simulink model "gm_sampleModel61741_pp_47_1_sub"  (R2023b)
settings: Solver=VariableStepAuto  StartTime=0.0  StopTime=10.0  RelTol=1e-3
libraries: simulink x46, hdlsllib x1
(part 1 of 2)
settings Model: Creator=CW  LastModifiedBy=CW
settings OptimizationCC: BlockReduction=off  ConditionallyExecuteInputs=off
settings DebuggingCC: ArtificialAlgebraicLoopMsg=none  InheritedTsInSrcMsg=none

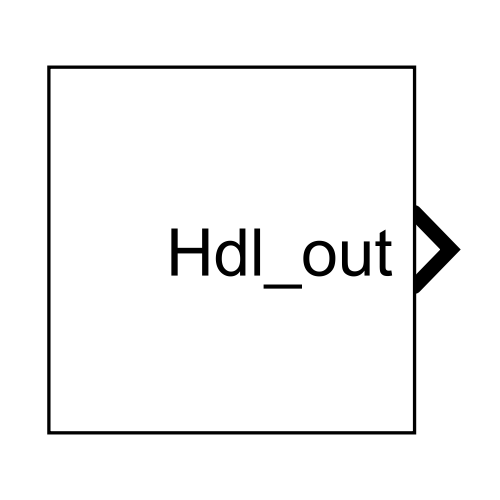
[thumbnail: Simulink's stored preview of the top-level diagram]
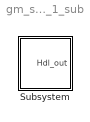
== system gm_sampleModel61741_pp_47_1_sub ==
  Subsystem : Subsystem

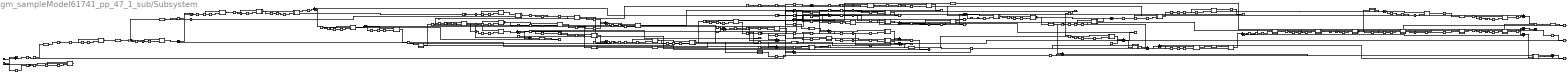
== system gm_sampleModel61741_pp_47_1_sub/Subsystem ==
  Reshape{,1..5} (6 alike) : Reshape
  cfblk1 : Subsystem  mask(Compare To Constant){relop=<=, const=double(3), OutDataTypeStr=uint8, ZeroCross=on}
      mask prompts: relop "Simulink:masks:Operator_MP"; const "Simulink:masks:ConstantValue_MP"; OutDataTypeStr "Simulink:masks:OutputDataType_MP"; ZeroCross "Simulink:masks:EnableZerocrossingDetection_MP"
      mask help: Simulink:masks:CompareToConstant_MD
      mask init:
      | OutDataTypeStr = 'uint8';
      | ZeroCross = 'on';
      | blkName = 'sampleModel61741_pp_47_1_sub/Subsystem/cfblk1';
      | const = double(3);
      | const_str = '3.0';
      | const_val = double(3);
      | relop = '<=';
      | setValue = 'fixdt(0, 8)';
      | str = '<= 3';
      mask TypeOptions relop: == | ~= | < | <= | >= | >
      mask TypeOptions OutDataTypeStr: Simulink:masks:uint8 | Simulink:masks:boolean
      mask Callback ZeroCross: sl('zeroCrossEnable', gcbh);
      mask Display: disp(str)
  cfblk{7,10,21,43,59,74,90,100,104,112,115,118,138,140,144,148} (16 alike) : Sum  OutDataTypeStr=uint8  AccumDataTypeStr=uint8  SampleTime=1
  cfblk{37,68,101,146} (4 alike) : MinMax  OutDataTypeStr=uint8
  cfblk{15..16,36,47,95,102,106,125,147} (9 alike) : Abs  SampleTime=1  OutDataTypeStr=uint8  SaturateOnIntegerOverflow=off
  cfblk103 : Subsystem
  cfblk{58,85,92,105} (4 alike) : Signum  SampleTime=1
  cfblk{18,73,93..94,107,131,145} (7 alike) : Sum  OutDataTypeStr=uint8  AccumDataTypeStr=uint8  RndMeth=Nearest  SampleTime=1
  cfblk107_const_val : Constant  Value=0  VectorParams1D=off  OutDataTypeStr=uint8  SampleTime=1
  cfblk109_inst : Subsystem
  cfblk11 : Sum  Inputs=+  OutDataTypeStr=uint8
  cfblk{22,27,39,44,61,69,86,110,128,137} (10 alike) : Sum  Inputs=+-  OutDataTypeStr=uint8  AccumDataTypeStr=uint8  SampleTime=1
  cfblk111 : Subsystem
  cfblk113 : Subsystem
  cfblk{20,24,35,54,57,91,114,134} (8 alike) : ComplexToRealImag  SampleTime=1
  cfblk{6,30,40,42,46,67,72,79..80,97,117,119,123} (13 alike) : Product  Inputs=*/  OutDataTypeStr=uint8  RndMeth=Zero  SaturateOnIntegerOverflow=on  SampleTime=1
  cfblk12 : Subsystem
  cfblk121 : Subsystem
  cfblk122 : Subsystem
  cfblk124 : Sum  Inputs=+  OutDataTypeStr=uint8
  cfblk126 : Subsystem  mask(Real World Value Increment){}
      mask help: Simulink:masks:RealWorldValueIncrement_MD
      mask Display: disp('V++')
  cfblk127 : Subsystem  mask(Real World Value Increment){}
      mask help: Simulink:masks:RealWorldValueIncrement_MD
      mask Display: disp('V++')
  cfblk13 : Subsystem
  cfblk130 : Subsystem
  cfblk131_const_val : Constant  Value=0  VectorParams1D=off  OutDataTypeStr=uint8  SampleTime=1
  cfblk132 : Subsystem
  cfblk133 : Subsystem
  cfblk135 : Subsystem
  cfblk139 : Subsystem
  cfblk14 : Subsystem
  cfblk141 : Subsystem  mask(Real World Value Increment){}
      mask help: Simulink:masks:RealWorldValueIncrement_MD
      mask Display: disp('V++')
  cfblk142 : Subsystem
  cfblk143_inst : Subsystem
  cfblk145_const_val : Constant  Value=0  VectorParams1D=off  OutDataTypeStr=uint8  SampleTime=1
  cfblk151 : Constant  OutDataTypeStr=uint8  SampleTime=1
  cfblk152 : Constant  OutDataTypeStr=uint8  SampleTime=1
  cfblk153 : hdlsllib/Sources/HDL Counter  CountType=Count limited  CountInit=0  CountStep=1  CountMax=25  CountFromType=Initial value  CountFrom=0  CountResetPort=off  CountLoadPort=off  CountEnbPort=off  CountDirPort=off  CountHitOutputPort=off  CountDataType=Unsigned  CountWordLen=8  CountFracLen=0  CountSampTime=1
  cfblk154 : Subsystem
  cfblk155 : Subsystem
  cfblk156 : Subsystem
  cfblk{157..160,162..171} (14 alike) : Delay  DelayLength=double(2)  InitialCondition=0  SampleTime=1
  cfblk17 : Gain  Gain="fi(0,0,8,7,\"hex\",\"80\")"  ParamDataTypeStr=fixdt(0, 8, 7)  OutDataTypeStr=uint8  SampleTime=1
  cfblk172 : Subsystem
  cfblk173 : DataTypeConversion  OutDataTypeStr=fixdt(0,8,0)
  cfblk174 : DataTypeConversion  OutDataTypeStr=fixdt(0,8,0)
  cfblk175 : Subsystem
  cfblk176 : Subsystem
  cfblk177 : Subsystem
  cfblk178 : DataTypeConversion  OutDataTypeStr=fixdt(0,8,0)
  cfblk18_const_val : Constant  Value=0  VectorParams1D=off  OutDataTypeStr=uint8  SampleTime=1
  cfblk19 : Subsystem
  cfblk2 : Subsystem  mask(Compare To Constant){relop=<=, const=double(3), OutDataTypeStr=uint8, ZeroCross=on}
      mask prompts: relop "Simulink:masks:Operator_MP"; const "Simulink:masks:ConstantValue_MP"; OutDataTypeStr "Simulink:masks:OutputDataType_MP"; ZeroCross "Simulink:masks:EnableZerocrossingDetection_MP"
      mask help: Simulink:masks:CompareToConstant_MD
      mask init:
      | OutDataTypeStr = 'uint8';
      | ZeroCross = 'on';
      | blkName = 'sampleModel61741_pp_47_1_sub/Subsystem/cfblk2';
      | const = double(3);
      | const_str = '3.0';
      | const_val = double(3);
      | relop = '<=';
      | setValue = 'fixdt(0, 8)';
      | str = '<= 3';
      mask TypeOptions relop: == | ~= | < | <= | >= | >
      mask TypeOptions OutDataTypeStr: Simulink:masks:uint8 | Simulink:masks:boolean
      mask Callback ZeroCross: sl('zeroCrossEnable', gcbh);
      mask Display: disp(str)
  cfblk23 : Subsystem
  cfblk26 : Subsystem
  cfblk28 : Subsystem
  cfblk29 : Sum  Inputs=+  OutDataTypeStr=uint8
  cfblk3 : simulink/Logic and Bit Operations/Detect Change  vinit=0  OutDataTypeStr=uint8
      settings: LibrarySourceBlock=|
      | hdlsllib/Logic and Bit
      | Operations/Detect
      | Change
  cfblk31_inst : Subsystem
  cfblk32 : Subsystem
  cfblk33 : Subsystem
  cfblk34 : Subsystem  mask(Real World Value Increment){}
      mask help: Simulink:masks:RealWorldValueIncrement_MD
      mask Display: disp('V++')
  cfblk38 : Subsystem  mask(Real World Value Increment){}
      mask help: Simulink:masks:RealWorldValueIncrement_MD
      mask Display: disp('V++')
  cfblk4 : Subsystem  mask(Detect Rise Nonnegative){vinit=double(0), InputProcessing=Elements as channels (sample based), OutDataTypeStr=uint8}
      mask prompts: vinit "Simulink:masks:InitialCondition_MP"; InputProcessing "Simulink:masks:InputProcessing_MP"; OutDataTypeStr "Simulink:masks:OutputDataType_MP"
      mask help: Simulink:masks:DetectRiseNonnegative_MD
      mask init:
      | InputProcessing = 'Elements as channels (sample based)';
      | OutDataTypeStr = 'uint8';
      | vinit = double(0);
      mask TypeOptions InputProcessing: Simulink:masks:ColumnsAsChannelsFrameBased | Simulink:masks:ElementsAsChannelsSampleBased
      mask TypeOptions OutDataTypeStr: Simulink:masks:uint8 | Simulink:masks:boolean
      mask Display: fprintf('U >= 0\n&  NOT\nU/z >= 0')
  cfblk41 : Subsystem
  cfblk45 : Subsystem  mask(Real World Value Increment){}
      mask help: Simulink:masks:RealWorldValueIncrement_MD
      mask Display: disp('V++')
  cfblk48 : Subsystem
  cfblk49 : Subsystem  mask(Real World Value Increment){}
      mask help: Simulink:masks:RealWorldValueIncrement_MD
      mask Display: disp('V++')
  cfblk5 : simulink/Logic and Bit Operations/Detect Decrease  vinit=0.0  OutDataTypeStr=uint8
      settings: LibrarySourceBlock=|
      | hdlsllib/Logic and Bit
      | Operations/Detect
      | Decrease
  cfblk50_inst : Subsystem
  cfblk51 : Subsystem
  cfblk55 : Subsystem
  cfblk56 : Subsystem
  cfblk60 : Subsystem
  cfblk62 : Subsystem
  cfblk63 : Subsystem  mask(Real World Value Increment){}
      mask help: Simulink:masks:RealWorldValueIncrement_MD
      mask Display: disp('V++')
  cfblk64 : Subsystem
  cfblk65 : Subsystem
  cfblk66 : Subsystem
  cfblk71 : Subsystem
  cfblk73_const_val : Constant  Value=0  VectorParams1D=off  OutDataTypeStr=uint8  SampleTime=1
  cfblk75 : Subsystem  mask(Real World Value Increment){}
      mask help: Simulink:masks:RealWorldValueIncrement_MD
      mask Display: disp('V++')
  cfblk76 : Subsystem
  cfblk77 : Subsystem
  cfblk78 : Subsystem
  cfblk8 : Subsystem
  cfblk81 : Subsystem
  cfblk82 : Subsystem
  cfblk83_inst : Subsystem
  cfblk87 : Subsystem
  cfblk9 : Gain  Gain="fi(0,0,8,7,\"hex\",\"80\")"  ParamDataTypeStr=fixdt(0, 8, 7)  OutDataTypeStr=uint8  SampleTime=1
  cfblk93_const_val : Constant  Value=0  VectorParams1D=off  OutDataTypeStr=uint8  SampleTime=1
  cfblk94_const_val : Constant  Value=0  VectorParams1D=off  OutDataTypeStr=uint8  SampleTime=1
  cfblk96_inst : Subsystem
  cfblk98 : Subsystem
  cfblk99 : Gain  Gain="fi(0,0,8,7,\"hex\",\"80\")"  ParamDataTypeStr=fixdt(0, 8, 7)  OutDataTypeStr=uint8  SampleTime=1
  compare{,2,7..8,14..16,23,25,32..33,35..36} (13 alike) : simulink/Logic and Bit Operations/Compare To Constant  relop=>=  const=0  OutDataTypeStr=boolean
  compare{1,3..4,6,9..13,17..20,22,26..27,30..31,34,37..38,40,42..43} (24 alike) : simulink/Logic and Bit Operations/Compare To Constant  relop=>=  const=255  OutDataTypeStr=boolean
  compare21 : simulink/Logic and Bit Operations/Compare To Constant  relop=>=  const=3  OutDataTypeStr=boolean
  compare24 : simulink/Logic and Bit Operations/Compare To Constant  relop=>=  const=2  OutDataTypeStr=boolean
  compare28 : simulink/Logic and Bit Operations/Compare To Constant  relop=>=  const=3  OutDataTypeStr=boolean
  compare{5,29,39,41} (4 alike) : simulink/Logic and Bit Operations/Compare To Constant  relop=>=  const=1  OutDataTypeStr=boolean
  emi_{6,14,23,31,39,47,55,63,71,79,87,95,103,111,120,128,136,144,152,161,169,177,186,194,202,210,218,227,235,244,252,261,269,277,285,293,309,317,325,333,341,349,357,365} (44 alike) : DataTypeConversion  OutDataTypeStr=fixdt(0,8,0)
  emi_{24,40,48,104,121,153,162,211,219,278,294,350,358} (13 alike) : Delay  DelayLength=double(2)  InitialCondition=0  SampleTime=1
  emi_{7,15,32,56,72,88,96,112,129,145,170,178,187,195,203,228,236,245,253,270,310,334,342,366} (24 alike) : Delay  DelayLength=double(2)  InitialCondition=255  SampleTime=1
  emi_{64,80,137,326} (4 alike) : Delay  DelayLength=double(2)  InitialCondition=1  SampleTime=1
  emi_262 : Delay  DelayLength=double(2)  InitialCondition=3  SampleTime=1
  emi_286 : Delay  DelayLength=double(2)  InitialCondition=2  SampleTime=1
  emi_318 : Delay  DelayLength=double(2)  InitialCondition=3  SampleTime=1
  Hdl_out : Outport  OutDataTypeStr=uint8  SampleTime=1
  wires:
  cfblk1/1(y) -> cfblk17/1
  cfblk10/1 -> cfblk22/1, cfblk80/2
  cfblk100/1 -> Hdl_out/1, cfblk155/1(In1)
  cfblk101/1 -> cfblk140/2
  cfblk102/1 -> emi_245/1, cfblk55/1(emi_238)
  cfblk103/1(emi_2) -> cfblk10/2
  cfblk104/1 -> cfblk138/2, cfblk115/1
  cfblk105/1 -> cfblk90/2, emi_112/1, cfblk139/1(emi_106)
  cfblk106/1 -> emi_278/1, cfblk172/1(emi_272)
  cfblk107/1 -> Reshape5/1
  cfblk109_inst/1(out1) -> cfblk148/2
  cfblk11/1 -> cfblk75/1(u)
  cfblk110/1 -> cfblk119/1
  cfblk111/1(emi_156) -> cfblk163/1
  cfblk111/2(emi_157) -> cfblk69/1, cfblk167/1
  cfblk112/1 -> emi_318/1, cfblk76/1(emi_312)
  cfblk113/1(emi_18) -> cfblk110/1
  cfblk113/2(emi_19) -> cfblk100/1
  cfblk114/1 -> cfblk5/1
  cfblk114/2 -> cfblk109_inst/1(in1)
  cfblk115/1 -> cfblk74/2
  Reshape/1 -> emi_342/1, cfblk82/1(emi_336)
  cfblk117/1 -> cfblk128/2, cfblk102/1, cfblk100/2
  cfblk118/1 -> emi_162/1, cfblk111/1(emi_155)
  cfblk119/1 -> cfblk162/1
  cfblk12/1(emi_35) -> emi_24/1, cfblk113/1(emi_17)
  Reshape1/1 -> emi_104/1, cfblk135/1(emi_98)
  cfblk121/1(emi_43) -> cfblk118/1
  cfblk122/1(emi_51) -> emi_145/1, cfblk98/1(emi_139)
  cfblk123/1 -> cfblk93/1
  cfblk124/1 -> cfblk72/2
  cfblk125/1 -> emi_170/1, cfblk19/1(emi_164), cfblk97/2
  cfblk126/1(y) -> cfblk86/1
  cfblk127/1(y) -> cfblk85/1, cfblk117/2
  cfblk128/1 -> emi_72/1, cfblk13/1(emi_66)
  cfblk13/1(emi_67) -> cfblk110/2
  cfblk130/1(emi_75) -> emi_137/1, cfblk175/1(emi_131)
  cfblk131/1 -> cfblk104/2, emi_326/1, cfblk78/1(emi_320)
  cfblk132/1(emi_83) -> emi_129/1, cfblk142/1(emi_123)
  cfblk133/1(emi_91) -> emi_270/1, cfblk62/1(emi_264)
  cfblk134/1 -> cfblk21/1
  cfblk134/2 -> cfblk90/1
  cfblk135/1(emi_99) -> cfblk44/2
  cfblk137/1 -> emi_334/1, cfblk8/1(emi_328)
  cfblk138/1 -> cfblk123/2
  cfblk139/1(emi_107) -> emi_253/1, cfblk56/1(emi_247)
  cfblk14/1(emi_115) -> cfblk173/1
  cfblk14/2(emi_116) -> cfblk174/1
  cfblk140/1 -> emi_178/1, cfblk23/1(emi_172)
  cfblk141/1(y) -> cfblk128/1
  cfblk142/1(emi_124) -> cfblk38/1(u), cfblk42/2
  cfblk143_inst/1(out1) -> cfblk59/1
  cfblk144/1 -> cfblk97/1
  cfblk145/1 -> cfblk95/1
  cfblk146/1 -> cfblk115/2
  cfblk147/1 -> cfblk165/1
  cfblk148/1 -> cfblk159/1
  cfblk15/1 -> cfblk158/1
  cfblk151/1 -> cfblk24/1
  cfblk152/1 -> cfblk131/1
  cfblk153/1 -> cfblk43/2, cfblk43/1, Reshape1/1
  cfblk154/1(emi_361) -> cfblk105/1
  cfblk155/1(Out1) -> Reshape2/1
  cfblk156/1(Out1) -> cfblk143_inst/1(in1)
  cfblk157/1 -> cfblk40/2
  cfblk158/1 -> cfblk79/2
  cfblk159/1 -> cfblk39/1
  cfblk16/1 -> cfblk137/1
  cfblk160/1 -> cfblk59/2
  cfblk162/1 -> cfblk83_inst/2(in2)
  cfblk163/1 -> cfblk42/1
  cfblk164/1 -> cfblk27/1
  cfblk165/1 -> cfblk10/1
  cfblk166/1 -> cfblk118/2
  cfblk167/1 -> cfblk138/1
  cfblk168/1 -> cfblk61/2
  cfblk169/1 -> cfblk80/1
  cfblk17/1 -> emi_64/1, cfblk81/1(emi_58)
  cfblk170/1 -> cfblk7/1
  cfblk171/1 -> cfblk30/2
  cfblk172/1(emi_273) -> cfblk54/1
  cfblk173/1 -> cfblk7/2
  cfblk174/1 -> emi_211/1, cfblk177/1(emi_205)
  cfblk175/1(emi_132) -> emi_121/1, cfblk14/1(emi_114)
  cfblk176/1(emi_148) -> cfblk67/2, cfblk29/1
  cfblk177/1(emi_206) -> cfblk50_inst/1(in1)
  cfblk178/1 -> cfblk50_inst/2(in2)
  cfblk18/1 -> cfblk148/1
  cfblk19/1(emi_165) -> cfblk134/1
  cfblk2/1(y) -> cfblk157/1
  cfblk20/1 -> Reshape3/1
  cfblk20/2 -> cfblk169/1, cfblk46/2
  cfblk21/1 -> cfblk44/1
  cfblk22/1 -> cfblk2/1(u)
  cfblk23/1(emi_173) -> cfblk127/1(u)
  cfblk24/1 -> cfblk35/1
  cfblk24/2 -> cfblk144/1
  Reshape2/1 -> cfblk96_inst/1(in1)
  cfblk26/1(emi_10) -> cfblk73/1
  cfblk27/1 -> emi_350/1, cfblk87/1(emi_344)
  cfblk28/1(emi_231) -> cfblk11/1
  cfblk29/1 -> cfblk140/1
  cfblk3/1 -> cfblk160/1
  cfblk30/1 -> cfblk57/1, emi_310/1, cfblk99/1, cfblk71/1(emi_304)
  cfblk31_inst/1(out1) -> cfblk168/1, cfblk6/2
  cfblk32/1(emi_181) -> cfblk171/1
  cfblk32/2(emi_182) -> cfblk69/2
  cfblk33/1(emi_353) -> emi_294/1, cfblk65/1(emi_288)
  cfblk34/1(y) -> cfblk18/1, cfblk9/1
  cfblk35/1 -> cfblk16/1
  cfblk35/2 -> cfblk36/1
  cfblk36/1 -> cfblk141/1(u)
  cfblk37/1 -> cfblk117/1
  cfblk38/1(y) -> cfblk146/1
  cfblk39/1 -> emi_195/1, cfblk41/1(emi_189)
  cfblk4/1(Y) -> cfblk178/1, cfblk124/1
  cfblk40/1 -> emi_32/1, cfblk77/1(emi_26)
  cfblk41/1(emi_190) -> cfblk156/1(In1)
  cfblk42/1 -> emi_228/1, cfblk51/1(emi_221)
  cfblk43/1 -> cfblk123/1
  cfblk44/1 -> cfblk15/1
  cfblk45/1(y) -> cfblk63/1(u)
  cfblk46/1 -> cfblk145/1
  cfblk47/1 -> cfblk144/2
  cfblk48/1(emi_214) -> cfblk1/1(u), cfblk4/1(U)
  cfblk49/1(y) -> cfblk21/2
  cfblk5/1 -> cfblk58/1
  cfblk50_inst/1(out1) -> emi_153/1, cfblk176/1(emi_147)
  cfblk51/1(emi_222) -> cfblk49/1(u)
  cfblk51/2(emi_223) -> cfblk20/1
  Reshape3/1 -> cfblk104/1, emi_40/1, cfblk12/1(emi_34)
  cfblk54/1 -> cfblk107/1
  cfblk54/2 -> cfblk68/1
  cfblk55/1(emi_239) -> cfblk170/1
  cfblk56/1(emi_248) -> emi_56/1, cfblk122/1(emi_50), cfblk126/1(u)
  cfblk57/1 -> cfblk31_inst/2(in2)
  cfblk57/2 -> cfblk22/2
  cfblk58/1 -> emi_219/1, cfblk48/1(emi_213)
  cfblk59/1 -> emi_366/1, cfblk154/1(emi_360)
  cfblk6/1 -> emi_203/1, cfblk66/1(emi_197)
  cfblk60/1(emi_256) -> cfblk92/1
  cfblk60/2(emi_257) -> cfblk86/2
  cfblk61/1 -> cfblk72/1
  cfblk62/1(emi_265) -> cfblk91/1
  cfblk63/1(y) -> cfblk46/1
  cfblk64/1(emi_281) -> cfblk112/2
  cfblk65/1(emi_289) -> cfblk112/1, cfblk34/1(u)
  cfblk66/1(emi_198) -> cfblk94/1
  cfblk67/1 -> emi_88/1, cfblk132/1(emi_82)
  cfblk68/1 -> cfblk106/1
  cfblk69/1 -> emi_358/1, cfblk33/1(emi_352)
  cfblk7/1 -> cfblk40/1
  cfblk71/1(emi_305) -> emi_96/1, emi_7/1, cfblk103/1(emi_1), cfblk133/1(emi_90)
  cfblk72/1 -> emi_80/1, cfblk130/1(emi_74)
  cfblk73/1 -> cfblk67/1
  cfblk74/1 -> cfblk39/2
  cfblk75/1(y) -> Reshape/1
  cfblk76/1(emi_313) -> Reshape4/1
  cfblk77/1(emi_27) -> cfblk27/2
  cfblk78/1(emi_321) -> cfblk37/1
  cfblk79/1 -> cfblk83_inst/1(in1)
  cfblk8/1(emi_329) -> emi_187/1, cfblk32/1(emi_180)
  cfblk80/1 -> emi_15/1, cfblk26/1(emi_9)
  cfblk81/1(emi_59) -> cfblk61/1
  cfblk82/1(emi_337) -> cfblk47/1
  cfblk83_inst/1(out1) -> cfblk30/1
  Reshape4/1 -> emi_262/1, cfblk60/1(emi_255)
  cfblk85/1 -> cfblk119/2
  cfblk86/1 -> emi_236/1, cfblk28/1(emi_230)
  cfblk87/1(emi_345) -> cfblk79/1
  Reshape5/1 -> cfblk114/1
  cfblk9/1 -> cfblk147/1, cfblk143_inst/2(in2), emi_286/1, cfblk64/1(emi_280), cfblk6/1
  cfblk90/1 -> cfblk109_inst/2(in2)
  cfblk91/1 -> cfblk101/1
  cfblk91/2 -> cfblk45/1(u)
  cfblk92/1 -> cfblk164/1
  cfblk93/1 -> emi_48/1, cfblk121/1(emi_42)
  cfblk94/1 -> cfblk96_inst/2(in2), cfblk166/1
  cfblk95/1 -> cfblk31_inst/1(in1)
  cfblk96_inst/1(out1) -> cfblk74/1
  cfblk97/1 -> cfblk3/1
  cfblk98/1(emi_140) -> cfblk125/1
  cfblk99/1 -> cfblk137/2
  emi_103/1 -> compare/1
  emi_104/1 -> emi_103/1
  emi_111/1 -> compare1/1
  emi_112/1 -> emi_111/1
  emi_120/1 -> compare2/1
  emi_121/1 -> emi_120/1
  emi_128/1 -> compare3/1
  emi_129/1 -> emi_128/1
  emi_136/1 -> compare5/1
  emi_137/1 -> emi_136/1
  emi_14/1 -> compare4/1
  emi_144/1 -> compare6/1
  emi_145/1 -> emi_144/1
  emi_15/1 -> emi_14/1
  emi_152/1 -> compare7/1
  emi_153/1 -> emi_152/1
  emi_161/1 -> compare8/1
  emi_162/1 -> emi_161/1
  emi_169/1 -> compare9/1
  emi_170/1 -> emi_169/1
  emi_177/1 -> compare10/1
  emi_178/1 -> emi_177/1
  emi_186/1 -> compare11/1
  emi_187/1 -> emi_186/1
  emi_194/1 -> compare12/1
  emi_195/1 -> emi_194/1
  emi_202/1 -> compare13/1
  emi_203/1 -> emi_202/1
  emi_210/1 -> compare14/1
  emi_211/1 -> emi_210/1
  emi_218/1 -> compare15/1
  emi_219/1 -> emi_218/1
  emi_227/1 -> compare17/1
  emi_228/1 -> emi_227/1
  emi_23/1 -> compare16/1
  emi_235/1 -> compare18/1
  emi_236/1 -> emi_235/1
  emi_24/1 -> emi_23/1
  emi_244/1 -> compare19/1
  emi_245/1 -> emi_244/1
  emi_252/1 -> compare20/1
  emi_253/1 -> emi_252/1
  emi_261/1 -> compare21/1
  emi_262/1 -> emi_261/1
  emi_269/1 -> compare22/1
  emi_270/1 -> emi_269/1
  emi_277/1 -> compare23/1
  emi_278/1 -> emi_277/1
  emi_285/1 -> compare24/1
  emi_286/1 -> emi_285/1
  emi_293/1 -> compare25/1
  emi_294/1 -> emi_293/1
  emi_309/1 -> compare27/1
  emi_31/1 -> compare26/1
  emi_310/1 -> emi_309/1
  emi_317/1 -> compare28/1
  emi_318/1 -> emi_317/1
  emi_32/1 -> emi_31/1
  emi_325/1 -> compare29/1
  emi_326/1 -> emi_325/1
  emi_333/1 -> compare30/1
  emi_334/1 -> emi_333/1
  emi_341/1 -> compare31/1
  emi_342/1 -> emi_341/1
  emi_349/1 -> compare32/1
  emi_350/1 -> emi_349/1
  emi_357/1 -> compare33/1
  emi_358/1 -> emi_357/1
  emi_365/1 -> compare34/1
  emi_366/1 -> emi_365/1
  emi_39/1 -> compare35/1
  emi_40/1 -> emi_39/1
  emi_47/1 -> compare36/1
  emi_48/1 -> emi_47/1
  emi_55/1 -> compare38/1
  emi_56/1 -> emi_55/1
  emi_6/1 -> compare37/1
  emi_63/1 -> compare39/1
  emi_64/1 -> emi_63/1
  emi_7/1 -> emi_6/1
  emi_71/1 -> compare40/1
  emi_72/1 -> emi_71/1
  emi_79/1 -> compare41/1
  emi_80/1 -> emi_79/1
  emi_87/1 -> compare42/1
  emi_88/1 -> emi_87/1
  emi_95/1 -> compare43/1
  emi_96/1 -> emi_95/1
  cfblk107_const_val/1 -> cfblk107/2
  cfblk131_const_val/1 -> cfblk131/2
  cfblk145_const_val/1 -> cfblk145/2
  cfblk18_const_val/1 -> cfblk18/2
  cfblk73_const_val/1 -> cfblk73/2
  cfblk93_const_val/1 -> cfblk93/2
  cfblk94_const_val/1 -> cfblk94/2
  compare/1 -> cfblk135/2(Action Port)
  compare1/1 -> cfblk139/2(Action Port)
  compare2/1 -> cfblk14/2(Action Port)
  compare3/1 -> cfblk142/2(Action Port)
  compare4/1 -> cfblk26/2(Action Port)
  compare5/1 -> cfblk175/2(Action Port)
  compare6/1 -> cfblk98/2(Action Port)
  compare7/1 -> cfblk176/2(Action Port)
  compare8/1 -> cfblk111/2(Action Port)
  compare9/1 -> cfblk19/2(Action Port)
  compare10/1 -> cfblk23/2(Action Port)
  compare11/1 -> cfblk32/2(Action Port)
  compare12/1 -> cfblk41/2(Action Port)
  compare13/1 -> cfblk66/2(Action Port)
  compare14/1 -> cfblk177/2(Action Port)
  compare15/1 -> cfblk48/2(Action Port)
  compare16/1 -> cfblk113/2(Action Port)
  compare17/1 -> cfblk51/2(Action Port)
  compare18/1 -> cfblk28/2(Action Port)
  compare19/1 -> cfblk55/2(Action Port)
  compare20/1 -> cfblk56/2(Action Port)
  compare21/1 -> cfblk60/2(Action Port)
  compare22/1 -> cfblk62/2(Action Port)
  compare23/1 -> cfblk172/2(Action Port)
  compare24/1 -> cfblk64/2(Action Port)
  compare25/1 -> cfblk65/2(Action Port)
  compare26/1 -> cfblk77/2(Action Port)
  compare27/1 -> cfblk71/2(Action Port)
  compare28/1 -> cfblk76/2(Action Port)
  compare29/1 -> cfblk78/2(Action Port)
  compare30/1 -> cfblk8/2(Action Port)
  compare31/1 -> cfblk82/2(Action Port)
  compare32/1 -> cfblk87/2(Action Port)
  compare33/1 -> cfblk33/2(Action Port)
  compare34/1 -> cfblk154/2(Action Port)
  compare35/1 -> cfblk12/2(Action Port)
  compare36/1 -> cfblk121/2(Action Port)
  compare37/1 -> cfblk103/2(Action Port)
  compare38/1 -> cfblk122/2(Action Port)
  compare39/1 -> cfblk81/2(Action Port)
  compare40/1 -> cfblk13/2(Action Port)
  compare41/1 -> cfblk130/2(Action Port)
  compare42/1 -> cfblk132/2(Action Port)
  compare43/1 -> cfblk133/2(Action Port)

== system gm_sampleModel61741_pp_47_1_sub/Subsystem/cfblk1 ==
  u : Inport  OutDataTypeStr=uint8  SampleTime=1
  Compare : RelationalOperator  Operator=<=  OutDataTypeStr=fixdt(0, 8)
  Constant : Constant  DisableCoverage=on  Value=const  OutDataTypeStr=Inherit: Inherit via back propagation  SampleTime=-1
  y : Outport  SampleTime=1
  wires:
  u/1 -> Compare/1
  Compare/1 -> y/1
  Constant/1 -> Compare/2

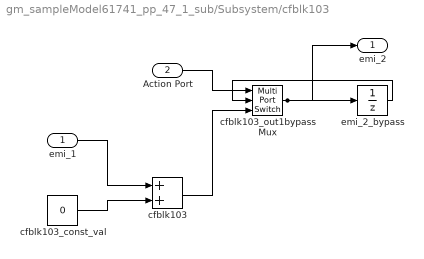
== system gm_sampleModel61741_pp_47_1_sub/Subsystem/cfblk103 ==
  emi_1 : Inport  OutDataTypeStr=uint8  PortDimensions=1  SampleTime=1
  Action Port : Inport  Port=2  OutDataTypeStr=boolean  SampleTime=1
  cfblk103 : Sum  OutDataTypeStr=uint8  AccumDataTypeStr=uint8  RndMeth=Nearest  SampleTime=1
  cfblk103_const_val : Constant  Value=0  VectorParams1D=off  OutDataTypeStr=uint8  SampleTime=1
  cfblk103_out1bypassMux : MultiPortSwitch  DataPortOrder=Zero-based contiguous  Inputs=2  zeroidx=on  OutDataTypeStr=uint8  SampleTime=1  SaturateOnIntegerOverflow=off  InputSameDT=off
  emi_2_bypass : UnitDelay  InitialCondition="fi(0,0,8,0,\"hex\",\"00\")"  SampleTime=1
  emi_2 : Outport  SampleTime=1  InitialOutput=0
  wires:
  Action Port/1 -> cfblk103_out1bypassMux/1
  emi_1/1 -> cfblk103/1
  cfblk103/1 -> cfblk103_out1bypassMux/3
  cfblk103_out1bypassMux/1 -> emi_2_bypass/1, emi_2/1
  emi_2_bypass/1 -> cfblk103_out1bypassMux/2
  cfblk103_const_val/1 -> cfblk103/2

== system gm_sampleModel61741_pp_47_1_sub/Subsystem/cfblk109_inst ==
  in1 : Inport  OutDataTypeStr=uint8  SampleTime=1
  in2 : Inport  Port=2  OutDataTypeStr=uint8  SampleTime=1
  mul_cfblk109_dotp_mulcomp : Product  Inputs=**  OutDataTypeStr=uint8  SampleTime=1
  out1 : Outport  OutDataTypeStr=uint8  SampleTime=1
  wires:
  in1/1 -> mul_cfblk109_dotp_mulcomp/1
  in2/1 -> mul_cfblk109_dotp_mulcomp/2
  mul_cfblk109_dotp_mulcomp/1 -> out1/1

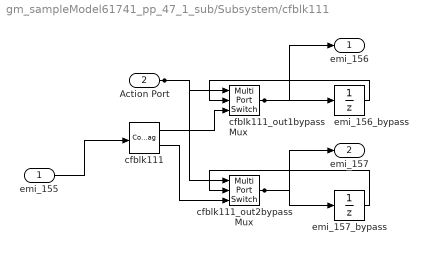
== system gm_sampleModel61741_pp_47_1_sub/Subsystem/cfblk111 ==
  emi_155 : Inport  OutDataTypeStr=uint8  PortDimensions=1  SampleTime=1
  Action Port : Inport  Port=2  OutDataTypeStr=boolean  SampleTime=1
  cfblk111 : ComplexToRealImag  SampleTime=1
  cfblk111_out1bypassMux : MultiPortSwitch  DataPortOrder=Zero-based contiguous  Inputs=2  zeroidx=on  OutDataTypeStr=uint8  SampleTime=1  SaturateOnIntegerOverflow=off  InputSameDT=off
  cfblk111_out2bypassMux : MultiPortSwitch  DataPortOrder=Zero-based contiguous  Inputs=2  zeroidx=on  OutDataTypeStr=uint8  SampleTime=1  SaturateOnIntegerOverflow=off  InputSameDT=off
  emi_156_bypass : UnitDelay  InitialCondition="fi(0,0,8,0,\"hex\",\"00\")"  SampleTime=1
  emi_157_bypass : UnitDelay  InitialCondition="fi(0,0,8,0,\"hex\",\"00\")"  SampleTime=1
  emi_156 : Outport  SampleTime=1  InitialOutput=0
  emi_157 : Outport  Port=2  SampleTime=1  InitialOutput=0
  wires:
  Action Port/1 -> cfblk111_out2bypassMux/1, cfblk111_out1bypassMux/1
  emi_155/1 -> cfblk111/1
  cfblk111/1 -> cfblk111_out1bypassMux/3
  cfblk111/2 -> cfblk111_out2bypassMux/3
  cfblk111_out1bypassMux/1 -> emi_156_bypass/1, emi_156/1
  emi_156_bypass/1 -> cfblk111_out1bypassMux/2
  cfblk111_out2bypassMux/1 -> emi_157_bypass/1, emi_157/1
  emi_157_bypass/1 -> cfblk111_out2bypassMux/2

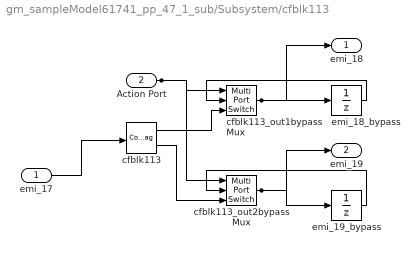
== system gm_sampleModel61741_pp_47_1_sub/Subsystem/cfblk113 ==
  emi_17 : Inport  OutDataTypeStr=uint8  PortDimensions=1  SampleTime=1
  Action Port : Inport  Port=2  OutDataTypeStr=boolean  SampleTime=1
  cfblk113 : ComplexToRealImag  SampleTime=1
  cfblk113_out1bypassMux : MultiPortSwitch  DataPortOrder=Zero-based contiguous  Inputs=2  zeroidx=on  OutDataTypeStr=uint8  SampleTime=1  SaturateOnIntegerOverflow=off  InputSameDT=off
  cfblk113_out2bypassMux : MultiPortSwitch  DataPortOrder=Zero-based contiguous  Inputs=2  zeroidx=on  OutDataTypeStr=uint8  SampleTime=1  SaturateOnIntegerOverflow=off  InputSameDT=off
  emi_18_bypass : UnitDelay  InitialCondition="fi(0,0,8,0,\"hex\",\"00\")"  SampleTime=1
  emi_19_bypass : UnitDelay  InitialCondition="fi(0,0,8,0,\"hex\",\"00\")"  SampleTime=1
  emi_18 : Outport  SampleTime=1  InitialOutput=0
  emi_19 : Outport  Port=2  SampleTime=1  InitialOutput=0
  wires:
  Action Port/1 -> cfblk113_out2bypassMux/1, cfblk113_out1bypassMux/1
  emi_17/1 -> cfblk113/1
  cfblk113/1 -> cfblk113_out1bypassMux/3
  cfblk113/2 -> cfblk113_out2bypassMux/3
  cfblk113_out1bypassMux/1 -> emi_18_bypass/1, emi_18/1
  emi_18_bypass/1 -> cfblk113_out1bypassMux/2
  cfblk113_out2bypassMux/1 -> emi_19_bypass/1, emi_19/1
  emi_19_bypass/1 -> cfblk113_out2bypassMux/2

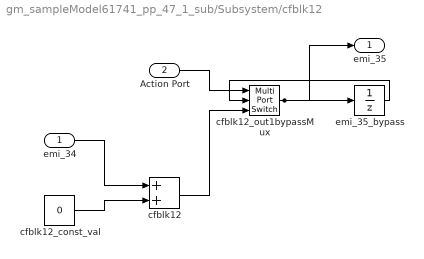
== system gm_sampleModel61741_pp_47_1_sub/Subsystem/cfblk12 ==
  emi_34 : Inport  OutDataTypeStr=uint8  PortDimensions=1  SampleTime=1
  Action Port : Inport  Port=2  OutDataTypeStr=boolean  SampleTime=1
  cfblk12 : Sum  OutDataTypeStr=uint8  AccumDataTypeStr=uint8  RndMeth=Nearest  SampleTime=1
  cfblk12_const_val : Constant  Value=0  VectorParams1D=off  OutDataTypeStr=uint8  SampleTime=1
  cfblk12_out1bypassMux : MultiPortSwitch  DataPortOrder=Zero-based contiguous  Inputs=2  zeroidx=on  OutDataTypeStr=uint8  SampleTime=1  SaturateOnIntegerOverflow=off  InputSameDT=off
  emi_35_bypass : UnitDelay  InitialCondition="fi(0,0,8,0,\"hex\",\"00\")"  SampleTime=1
  emi_35 : Outport  SampleTime=1  InitialOutput=0
  wires:
  Action Port/1 -> cfblk12_out1bypassMux/1
  emi_34/1 -> cfblk12/1
  cfblk12/1 -> cfblk12_out1bypassMux/3
  cfblk12_out1bypassMux/1 -> emi_35_bypass/1, emi_35/1
  emi_35_bypass/1 -> cfblk12_out1bypassMux/2
  cfblk12_const_val/1 -> cfblk12/2

== system gm_sampleModel61741_pp_47_1_sub/Subsystem/cfblk121 ==
  emi_42 : Inport  OutDataTypeStr=uint8  PortDimensions=1  SampleTime=1
  Action Port : Inport  Port=2  OutDataTypeStr=boolean  SampleTime=1
  Reshape : Reshape
  cfblk121_out1bypassMux : MultiPortSwitch  DataPortOrder=Zero-based contiguous  Inputs=2  zeroidx=on  OutDataTypeStr=uint8  SampleTime=1  SaturateOnIntegerOverflow=off  InputSameDT=off
  emi_43_bypass : UnitDelay  InitialCondition="fi(0,0,8,0,\"hex\",\"00\")"  SampleTime=1
  emi_43 : Outport  SampleTime=1  InitialOutput=0
  wires:
  Action Port/1 -> cfblk121_out1bypassMux/1
  emi_42/1 -> Reshape/1
  Reshape/1 -> cfblk121_out1bypassMux/3
  cfblk121_out1bypassMux/1 -> emi_43_bypass/1, emi_43/1
  emi_43_bypass/1 -> cfblk121_out1bypassMux/2

== system gm_sampleModel61741_pp_47_1_sub/Subsystem/cfblk122 ==
  emi_50 : Inport  OutDataTypeStr=uint8  PortDimensions=1  SampleTime=1
  Action Port : Inport  Port=2  OutDataTypeStr=boolean  SampleTime=1
  Reshape : Reshape
  cfblk122_out1bypassMux : MultiPortSwitch  DataPortOrder=Zero-based contiguous  Inputs=2  zeroidx=on  OutDataTypeStr=uint8  SampleTime=1  SaturateOnIntegerOverflow=off  InputSameDT=off
  emi_51_bypass : UnitDelay  InitialCondition="fi(0,0,8,0,\"hex\",\"00\")"  SampleTime=1
  emi_51 : Outport  SampleTime=1  InitialOutput=0
  wires:
  Action Port/1 -> cfblk122_out1bypassMux/1
  emi_50/1 -> Reshape/1
  Reshape/1 -> cfblk122_out1bypassMux/3
  cfblk122_out1bypassMux/1 -> emi_51_bypass/1, emi_51/1
  emi_51_bypass/1 -> cfblk122_out1bypassMux/2

== system gm_sampleModel61741_pp_47_1_sub/Subsystem/cfblk126 ==
  u : Inport  OutDataTypeStr=uint8  SampleTime=1
  FixPt Constant : Constant  DisableCoverage=on  OutDataTypeStr=Inherit: Inherit via back propagation  SampleTime=-1
  FixPt Data Type Duplicate : DataTypeDuplicate  DisableCoverage=on  NumInputPorts=3
  FixPt Sum1 : Sum  OutDataTypeStr=Inherit: Inherit via back propagation  InputSameDT=on  LockScale=on
  y : Outport  SampleTime=1
  wires:
  u/1 -> FixPt Sum1/1, FixPt Data Type Duplicate/2
  FixPt Constant/1 -> FixPt Sum1/2, FixPt Data Type Duplicate/3
  FixPt Sum1/1 -> FixPt Data Type Duplicate/1, y/1

== system gm_sampleModel61741_pp_47_1_sub/Subsystem/cfblk127 ==
  u : Inport  OutDataTypeStr=uint8  SampleTime=1
  FixPt Constant : Constant  DisableCoverage=on  OutDataTypeStr=Inherit: Inherit via back propagation  SampleTime=-1
  FixPt Data Type Duplicate : DataTypeDuplicate  DisableCoverage=on  NumInputPorts=3
  FixPt Sum1 : Sum  OutDataTypeStr=Inherit: Inherit via back propagation  InputSameDT=on  LockScale=on
  y : Outport  SampleTime=1
  wires:
  u/1 -> FixPt Sum1/1, FixPt Data Type Duplicate/2
  FixPt Constant/1 -> FixPt Sum1/2, FixPt Data Type Duplicate/3
  FixPt Sum1/1 -> FixPt Data Type Duplicate/1, y/1

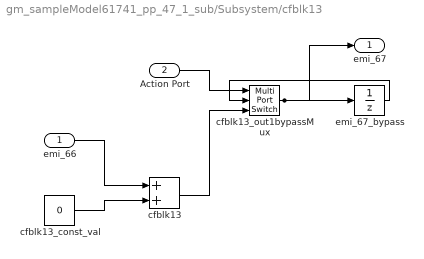
== system gm_sampleModel61741_pp_47_1_sub/Subsystem/cfblk13 ==
  emi_66 : Inport  OutDataTypeStr=uint8  PortDimensions=1  SampleTime=1
  Action Port : Inport  Port=2  OutDataTypeStr=boolean  SampleTime=1
  cfblk13 : Sum  OutDataTypeStr=uint8  AccumDataTypeStr=uint8  RndMeth=Nearest  SampleTime=1
  cfblk13_const_val : Constant  Value=0  VectorParams1D=off  OutDataTypeStr=uint8  SampleTime=1
  cfblk13_out1bypassMux : MultiPortSwitch  DataPortOrder=Zero-based contiguous  Inputs=2  zeroidx=on  OutDataTypeStr=uint8  SampleTime=1  SaturateOnIntegerOverflow=off  InputSameDT=off
  emi_67_bypass : UnitDelay  InitialCondition="fi(0,0,8,0,\"hex\",\"00\")"  SampleTime=1
  emi_67 : Outport  SampleTime=1  InitialOutput=0
  wires:
  Action Port/1 -> cfblk13_out1bypassMux/1
  emi_66/1 -> cfblk13/1
  cfblk13/1 -> cfblk13_out1bypassMux/3
  cfblk13_out1bypassMux/1 -> emi_67_bypass/1, emi_67/1
  emi_67_bypass/1 -> cfblk13_out1bypassMux/2
  cfblk13_const_val/1 -> cfblk13/2

== system gm_sampleModel61741_pp_47_1_sub/Subsystem/cfblk130 ==
  emi_74 : Inport  OutDataTypeStr=uint8  PortDimensions=1  SampleTime=1
  Action Port : Inport  Port=2  OutDataTypeStr=boolean  SampleTime=1
  cfblk130 : Signum  SampleTime=1
  cfblk130_out1bypassMux : MultiPortSwitch  DataPortOrder=Zero-based contiguous  Inputs=2  zeroidx=on  OutDataTypeStr=uint8  SampleTime=1  SaturateOnIntegerOverflow=off  InputSameDT=off
  emi_75_bypass : UnitDelay  InitialCondition="fi(0,0,8,0,\"hex\",\"00\")"  SampleTime=1
  emi_75 : Outport  SampleTime=1  InitialOutput=0
  wires:
  Action Port/1 -> cfblk130_out1bypassMux/1
  emi_74/1 -> cfblk130/1
  cfblk130/1 -> cfblk130_out1bypassMux/3
  cfblk130_out1bypassMux/1 -> emi_75_bypass/1, emi_75/1
  emi_75_bypass/1 -> cfblk130_out1bypassMux/2

== system gm_sampleModel61741_pp_47_1_sub/Subsystem/cfblk132 ==
  emi_82 : Inport  OutDataTypeStr=uint8  PortDimensions=1  SampleTime=1
  Action Port : Inport  Port=2  OutDataTypeStr=boolean  SampleTime=1
  Reshape : Reshape
  cfblk132_out1bypassMux : MultiPortSwitch  DataPortOrder=Zero-based contiguous  Inputs=2  zeroidx=on  OutDataTypeStr=uint8  SampleTime=1  SaturateOnIntegerOverflow=off  InputSameDT=off
  emi_83_bypass : UnitDelay  InitialCondition="fi(0,0,8,0,\"hex\",\"00\")"  SampleTime=1
  emi_83 : Outport  SampleTime=1  InitialOutput=0
  wires:
  Action Port/1 -> cfblk132_out1bypassMux/1
  emi_82/1 -> Reshape/1
  Reshape/1 -> cfblk132_out1bypassMux/3
  cfblk132_out1bypassMux/1 -> emi_83_bypass/1, emi_83/1
  emi_83_bypass/1 -> cfblk132_out1bypassMux/2

== system gm_sampleModel61741_pp_47_1_sub/Subsystem/cfblk133 ==
  emi_90 : Inport  OutDataTypeStr=uint8  PortDimensions=1  SampleTime=1
  Action Port : Inport  Port=2  OutDataTypeStr=boolean  SampleTime=1
  cfblk133 : Signum  SampleTime=1
  cfblk133_out1bypassMux : MultiPortSwitch  DataPortOrder=Zero-based contiguous  Inputs=2  zeroidx=on  OutDataTypeStr=uint8  SampleTime=1  SaturateOnIntegerOverflow=off  InputSameDT=off
  emi_91_bypass : UnitDelay  InitialCondition="fi(0,0,8,0,\"hex\",\"00\")"  SampleTime=1
  emi_91 : Outport  SampleTime=1  InitialOutput=0
  wires:
  Action Port/1 -> cfblk133_out1bypassMux/1
  emi_90/1 -> cfblk133/1
  cfblk133/1 -> cfblk133_out1bypassMux/3
  cfblk133_out1bypassMux/1 -> emi_91_bypass/1, emi_91/1
  emi_91_bypass/1 -> cfblk133_out1bypassMux/2

== system gm_sampleModel61741_pp_47_1_sub/Subsystem/cfblk135 ==
  emi_98 : Inport  OutDataTypeStr=uint8  PortDimensions=1  SampleTime=1
  Action Port : Inport  Port=2  OutDataTypeStr=boolean  SampleTime=1
  Reshape : Reshape
  cfblk135_out1bypassMux : MultiPortSwitch  DataPortOrder=Zero-based contiguous  Inputs=2  zeroidx=on  OutDataTypeStr=uint8  SampleTime=1  SaturateOnIntegerOverflow=off  InputSameDT=off
  emi_99_bypass : UnitDelay  InitialCondition="fi(0,0,8,0,\"hex\",\"00\")"  SampleTime=1
  emi_99 : Outport  SampleTime=1  InitialOutput=0
  wires:
  Action Port/1 -> cfblk135_out1bypassMux/1
  emi_98/1 -> Reshape/1
  Reshape/1 -> cfblk135_out1bypassMux/3
  cfblk135_out1bypassMux/1 -> emi_99_bypass/1, emi_99/1
  emi_99_bypass/1 -> cfblk135_out1bypassMux/2

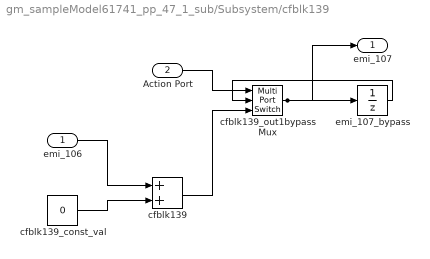
== system gm_sampleModel61741_pp_47_1_sub/Subsystem/cfblk139 ==
  emi_106 : Inport  OutDataTypeStr=uint8  PortDimensions=1  SampleTime=1
  Action Port : Inport  Port=2  OutDataTypeStr=boolean  SampleTime=1
  cfblk139 : Sum  OutDataTypeStr=uint8  AccumDataTypeStr=uint8  RndMeth=Nearest  SampleTime=1
  cfblk139_const_val : Constant  Value=0  VectorParams1D=off  OutDataTypeStr=uint8  SampleTime=1
  cfblk139_out1bypassMux : MultiPortSwitch  DataPortOrder=Zero-based contiguous  Inputs=2  zeroidx=on  OutDataTypeStr=uint8  SampleTime=1  SaturateOnIntegerOverflow=off  InputSameDT=off
  emi_107_bypass : UnitDelay  InitialCondition="fi(0,0,8,0,\"hex\",\"00\")"  SampleTime=1
  emi_107 : Outport  SampleTime=1  InitialOutput=0
  wires:
  Action Port/1 -> cfblk139_out1bypassMux/1
  emi_106/1 -> cfblk139/1
  cfblk139/1 -> cfblk139_out1bypassMux/3
  cfblk139_out1bypassMux/1 -> emi_107_bypass/1, emi_107/1
  emi_107_bypass/1 -> cfblk139_out1bypassMux/2
  cfblk139_const_val/1 -> cfblk139/2

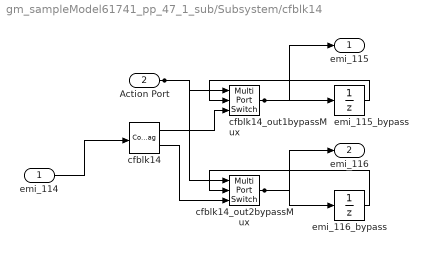
== system gm_sampleModel61741_pp_47_1_sub/Subsystem/cfblk14 ==
  emi_114 : Inport  OutDataTypeStr=uint8  PortDimensions=1  SampleTime=1
  Action Port : Inport  Port=2  OutDataTypeStr=boolean  SampleTime=1
  cfblk14 : ComplexToRealImag  SampleTime=1
  cfblk14_out1bypassMux : MultiPortSwitch  DataPortOrder=Zero-based contiguous  Inputs=2  zeroidx=on  OutDataTypeStr=uint8  SampleTime=1  SaturateOnIntegerOverflow=off  InputSameDT=off
  cfblk14_out2bypassMux : MultiPortSwitch  DataPortOrder=Zero-based contiguous  Inputs=2  zeroidx=on  OutDataTypeStr=uint8  SampleTime=1  SaturateOnIntegerOverflow=off  InputSameDT=off
  emi_115_bypass : UnitDelay  InitialCondition="fi(0,0,8,0,\"hex\",\"00\")"  SampleTime=1
  emi_116_bypass : UnitDelay  InitialCondition="fi(0,0,8,0,\"hex\",\"00\")"  SampleTime=1
  emi_115 : Outport  SampleTime=1  InitialOutput=0
  emi_116 : Outport  Port=2  SampleTime=1  InitialOutput=0
  wires:
  Action Port/1 -> cfblk14_out2bypassMux/1, cfblk14_out1bypassMux/1
  emi_114/1 -> cfblk14/1
  cfblk14/1 -> cfblk14_out1bypassMux/3
  cfblk14/2 -> cfblk14_out2bypassMux/3
  cfblk14_out1bypassMux/1 -> emi_115_bypass/1, emi_115/1
  emi_115_bypass/1 -> cfblk14_out1bypassMux/2
  cfblk14_out2bypassMux/1 -> emi_116_bypass/1, emi_116/1
  emi_116_bypass/1 -> cfblk14_out2bypassMux/2

== system gm_sampleModel61741_pp_47_1_sub/Subsystem/cfblk141 ==
  u : Inport  OutDataTypeStr=uint8  SampleTime=1
  FixPt Constant : Constant  DisableCoverage=on  OutDataTypeStr=Inherit: Inherit via back propagation  SampleTime=-1
  FixPt Data Type Duplicate : DataTypeDuplicate  DisableCoverage=on  NumInputPorts=3
  FixPt Sum1 : Sum  OutDataTypeStr=Inherit: Inherit via back propagation  InputSameDT=on  LockScale=on
  y : Outport  SampleTime=1
  wires:
  u/1 -> FixPt Sum1/1, FixPt Data Type Duplicate/2
  FixPt Constant/1 -> FixPt Sum1/2, FixPt Data Type Duplicate/3
  FixPt Sum1/1 -> FixPt Data Type Duplicate/1, y/1

== system gm_sampleModel61741_pp_47_1_sub/Subsystem/cfblk142 ==
  emi_123 : Inport  OutDataTypeStr=uint8  PortDimensions=1  SampleTime=1
  Action Port : Inport  Port=2  OutDataTypeStr=boolean  SampleTime=1
  Reshape : Reshape
  cfblk142_out1bypassMux : MultiPortSwitch  DataPortOrder=Zero-based contiguous  Inputs=2  zeroidx=on  OutDataTypeStr=uint8  SampleTime=1  SaturateOnIntegerOverflow=off  InputSameDT=off
  emi_124_bypass : UnitDelay  InitialCondition="fi(0,0,8,0,\"hex\",\"00\")"  SampleTime=1
  emi_124 : Outport  SampleTime=1  InitialOutput=0
  wires:
  Action Port/1 -> cfblk142_out1bypassMux/1
  emi_123/1 -> Reshape/1
  Reshape/1 -> cfblk142_out1bypassMux/3
  cfblk142_out1bypassMux/1 -> emi_124_bypass/1, emi_124/1
  emi_124_bypass/1 -> cfblk142_out1bypassMux/2

== system gm_sampleModel61741_pp_47_1_sub/Subsystem/cfblk143_inst ==
  in1 : Inport  OutDataTypeStr=uint8  SampleTime=1
  in2 : Inport  Port=2  OutDataTypeStr=uint8  SampleTime=1
  mul_cfblk143_dotp_mulcomp : Product  Inputs=**  OutDataTypeStr=uint8  SampleTime=1
  out1 : Outport  OutDataTypeStr=uint8  SampleTime=1
  wires:
  in1/1 -> mul_cfblk143_dotp_mulcomp/1
  in2/1 -> mul_cfblk143_dotp_mulcomp/2
  mul_cfblk143_dotp_mulcomp/1 -> out1/1

== system gm_sampleModel61741_pp_47_1_sub/Subsystem/cfblk154 ==
  emi_360 : Inport  OutDataTypeStr=uint8  PortDimensions=1  SampleTime=1
  Action Port : Inport  Port=2  OutDataTypeStr=boolean  SampleTime=1
  cfblk154 : Subsystem
  cfblk154_out1bypassMux : MultiPortSwitch  DataPortOrder=Zero-based contiguous  Inputs=2  zeroidx=on  OutDataTypeStr=uint8  SampleTime=1  SaturateOnIntegerOverflow=off  InputSameDT=off
  emi_361_bypass : UnitDelay  InitialCondition="fi(0,0,8,0,\"hex\",\"00\")"  SampleTime=1
  emi_361 : Outport  SampleTime=1  InitialOutput=0
  wires:
  Action Port/1 -> cfblk154_out1bypassMux/1
  emi_360/1 -> cfblk154/1(In1)
  cfblk154/1(Out1) -> cfblk154_out1bypassMux/3
  cfblk154_out1bypassMux/1 -> emi_361_bypass/1, emi_361/1
  emi_361_bypass/1 -> cfblk154_out1bypassMux/2

== system gm_sampleModel61741_pp_47_1_sub/Subsystem/cfblk155 ==
  In1 : Inport  OutDataTypeStr=uint8  PortDimensions=1  SampleTime=1
  Out1 : Outport  SampleTime=1  InitialOutput=[0]
  wires:
  In1/1 -> Out1/1

== system gm_sampleModel61741_pp_47_1_sub/Subsystem/cfblk156 ==
  In1 : Inport  OutDataTypeStr=uint8  PortDimensions=1  SampleTime=1
  Out1 : Outport  SampleTime=1  InitialOutput=[0]
  wires:
  In1/1 -> Out1/1

== system gm_sampleModel61741_pp_47_1_sub/Subsystem/cfblk172 ==
  emi_272 : Inport  OutDataTypeStr=uint8  PortDimensions=1  SampleTime=1
  Action Port : Inport  Port=2  OutDataTypeStr=boolean  SampleTime=1
  cfblk172 : Subsystem
      settings: MinAlgLoopOccurrences=on
  emi_273 : Outport  SampleTime=1  InitialOutput=0
  wires:
  Action Port/1 -> cfblk172/Enable
  emi_272/1 -> cfblk172/1(in0)
  cfblk172/1(out0) -> emi_273/1

== system gm_sampleModel61741_pp_47_1_sub/Subsystem/cfblk175 ==
  emi_131 : Inport  OutDataTypeStr=uint8  PortDimensions=1  SampleTime=1
  Action Port : Inport  Port=2  OutDataTypeStr=boolean  SampleTime=1
  cfblk175 : DataTypeConversion  OutDataTypeStr=fixdt(0,8,0)
  cfblk175_out1bypassMux : MultiPortSwitch  DataPortOrder=Zero-based contiguous  Inputs=2  zeroidx=on  OutDataTypeStr=uint8  SampleTime=1  SaturateOnIntegerOverflow=off  InputSameDT=off
  emi_132_bypass : UnitDelay  InitialCondition="fi(0,0,8,0,\"hex\",\"00\")"  SampleTime=1
  emi_132 : Outport  SampleTime=1  InitialOutput=0
  wires:
  Action Port/1 -> cfblk175_out1bypassMux/1
  emi_131/1 -> cfblk175/1
  cfblk175/1 -> cfblk175_out1bypassMux/3
  cfblk175_out1bypassMux/1 -> emi_132_bypass/1, emi_132/1
  emi_132_bypass/1 -> cfblk175_out1bypassMux/2

== system gm_sampleModel61741_pp_47_1_sub/Subsystem/cfblk176 ==
  emi_147 : Inport  OutDataTypeStr=uint8  PortDimensions=1  SampleTime=1
  Action Port : Inport  Port=2  OutDataTypeStr=boolean  SampleTime=1
  cfblk176 : DataTypeConversion  OutDataTypeStr=fixdt(0,8,0)
  cfblk176_out1bypassMux : MultiPortSwitch  DataPortOrder=Zero-based contiguous  Inputs=2  zeroidx=on  OutDataTypeStr=uint8  SampleTime=1  SaturateOnIntegerOverflow=off  InputSameDT=off
  emi_148_bypass : UnitDelay  InitialCondition="fi(0,0,8,0,\"hex\",\"00\")"  SampleTime=1
  emi_148 : Outport  SampleTime=1  InitialOutput=0
  wires:
  Action Port/1 -> cfblk176_out1bypassMux/1
  emi_147/1 -> cfblk176/1
  cfblk176/1 -> cfblk176_out1bypassMux/3
  cfblk176_out1bypassMux/1 -> emi_148_bypass/1, emi_148/1
  emi_148_bypass/1 -> cfblk176_out1bypassMux/2

== system gm_sampleModel61741_pp_47_1_sub/Subsystem/cfblk177 ==
  emi_205 : Inport  OutDataTypeStr=uint8  PortDimensions=1  SampleTime=1
  Action Port : Inport  Port=2  OutDataTypeStr=boolean  SampleTime=1
  cfblk177 : DataTypeConversion  OutDataTypeStr=fixdt(0,8,0)
  cfblk177_out1bypassMux : MultiPortSwitch  DataPortOrder=Zero-based contiguous  Inputs=2  zeroidx=on  OutDataTypeStr=uint8  SampleTime=1  SaturateOnIntegerOverflow=off  InputSameDT=off
  emi_206_bypass : UnitDelay  InitialCondition="fi(0,0,8,0,\"hex\",\"00\")"  SampleTime=1
  emi_206 : Outport  SampleTime=1  InitialOutput=0
  wires:
  Action Port/1 -> cfblk177_out1bypassMux/1
  emi_205/1 -> cfblk177/1
  cfblk177/1 -> cfblk177_out1bypassMux/3
  cfblk177_out1bypassMux/1 -> emi_206_bypass/1, emi_206/1
  emi_206_bypass/1 -> cfblk177_out1bypassMux/2

== system gm_sampleModel61741_pp_47_1_sub/Subsystem/cfblk19 ==
  emi_164 : Inport  OutDataTypeStr=uint8  PortDimensions=1  SampleTime=1
  Action Port : Inport  Port=2  OutDataTypeStr=boolean  SampleTime=1
  cfblk19 : Sum  Inputs=+
  cfblk19_out1bypassMux : MultiPortSwitch  DataPortOrder=Zero-based contiguous  Inputs=2  zeroidx=on  OutDataTypeStr=uint8  SampleTime=1  SaturateOnIntegerOverflow=off  InputSameDT=off
  emi_165_bypass : UnitDelay  InitialCondition="fi(0,0,8,0,\"hex\",\"00\")"  SampleTime=1
  emi_165 : Outport  SampleTime=1  InitialOutput=0
  wires:
  Action Port/1 -> cfblk19_out1bypassMux/1
  emi_164/1 -> cfblk19/1
  cfblk19/1 -> cfblk19_out1bypassMux/3
  cfblk19_out1bypassMux/1 -> emi_165_bypass/1, emi_165/1
  emi_165_bypass/1 -> cfblk19_out1bypassMux/2

== system gm_sampleModel61741_pp_47_1_sub/Subsystem/cfblk2 ==
  u : Inport  OutDataTypeStr=uint8  SampleTime=1
  Compare : RelationalOperator  Operator=<=  OutDataTypeStr=fixdt(0, 8)
  Constant : Constant  DisableCoverage=on  Value=const  OutDataTypeStr=Inherit: Inherit via back propagation  SampleTime=-1
  y : Outport  SampleTime=1
  wires:
  u/1 -> Compare/1
  Compare/1 -> y/1
  Constant/1 -> Compare/2

== system gm_sampleModel61741_pp_47_1_sub/Subsystem/cfblk23 ==
  emi_172 : Inport  OutDataTypeStr=uint8  PortDimensions=1  SampleTime=1
  Action Port : Inport  Port=2  OutDataTypeStr=boolean  SampleTime=1
  cfblk23 : Abs  SampleTime=1  OutDataTypeStr=uint8  SaturateOnIntegerOverflow=off
  cfblk23_out1bypassMux : MultiPortSwitch  DataPortOrder=Zero-based contiguous  Inputs=2  zeroidx=on  OutDataTypeStr=uint8  SampleTime=1  SaturateOnIntegerOverflow=off  InputSameDT=off
  emi_173_bypass : UnitDelay  InitialCondition="fi(0,0,8,0,\"hex\",\"00\")"  SampleTime=1
  emi_173 : Outport  SampleTime=1  InitialOutput=0
  wires:
  Action Port/1 -> cfblk23_out1bypassMux/1
  emi_172/1 -> cfblk23/1
  cfblk23/1 -> cfblk23_out1bypassMux/3
  cfblk23_out1bypassMux/1 -> emi_173_bypass/1, emi_173/1
  emi_173_bypass/1 -> cfblk23_out1bypassMux/2

== system gm_sampleModel61741_pp_47_1_sub/Subsystem/cfblk26 ==
  emi_9 : Inport  OutDataTypeStr=uint8  PortDimensions=1  SampleTime=1
  Action Port : Inport  Port=2  OutDataTypeStr=boolean  SampleTime=1
  cfblk26 : MinMax
  cfblk26_out1bypassMux : MultiPortSwitch  DataPortOrder=Zero-based contiguous  Inputs=2  zeroidx=on  OutDataTypeStr=uint8  SampleTime=1  SaturateOnIntegerOverflow=off  InputSameDT=off
  emi_10_bypass : UnitDelay  InitialCondition="fi(0,0,8,0,\"hex\",\"00\")"  SampleTime=1
  emi_10 : Outport  SampleTime=1  InitialOutput=0
  wires:
  Action Port/1 -> cfblk26_out1bypassMux/1
  emi_9/1 -> cfblk26/1
  cfblk26/1 -> cfblk26_out1bypassMux/3
  cfblk26_out1bypassMux/1 -> emi_10_bypass/1, emi_10/1
  emi_10_bypass/1 -> cfblk26_out1bypassMux/2

== system gm_sampleModel61741_pp_47_1_sub/Subsystem/cfblk28 ==
  emi_230 : Inport  OutDataTypeStr=uint8  PortDimensions=1  SampleTime=1
  Action Port : Inport  Port=2  OutDataTypeStr=boolean  SampleTime=1
  cfblk28 : Sum  OutDataTypeStr=uint8  AccumDataTypeStr=uint8  RndMeth=Nearest  SampleTime=1
  cfblk28_const_val : Constant  Value=0  VectorParams1D=off  OutDataTypeStr=uint8  SampleTime=1
  cfblk28_out1bypassMux : MultiPortSwitch  DataPortOrder=Zero-based contiguous  Inputs=2  zeroidx=on  OutDataTypeStr=uint8  SampleTime=1  SaturateOnIntegerOverflow=off  InputSameDT=off
  emi_231_bypass : UnitDelay  InitialCondition="fi(0,0,8,0,\"hex\",\"00\")"  SampleTime=1
  emi_231 : Outport  SampleTime=1  InitialOutput=0
  wires:
  Action Port/1 -> cfblk28_out1bypassMux/1
  emi_230/1 -> cfblk28/1
  cfblk28/1 -> cfblk28_out1bypassMux/3
  cfblk28_out1bypassMux/1 -> emi_231_bypass/1, emi_231/1
  emi_231_bypass/1 -> cfblk28_out1bypassMux/2
  cfblk28_const_val/1 -> cfblk28/2

== system gm_sampleModel61741_pp_47_1_sub/Subsystem/cfblk31_inst ==
  in1 : Inport  OutDataTypeStr=uint8  SampleTime=1
  in2 : Inport  Port=2  OutDataTypeStr=uint8  SampleTime=1
  mul_cfblk31_dotp_mulcomp : Product  Inputs=**  OutDataTypeStr=uint8  SampleTime=1
  out1 : Outport  OutDataTypeStr=uint8  SampleTime=1
  wires:
  in1/1 -> mul_cfblk31_dotp_mulcomp/1
  in2/1 -> mul_cfblk31_dotp_mulcomp/2
  mul_cfblk31_dotp_mulcomp/1 -> out1/1

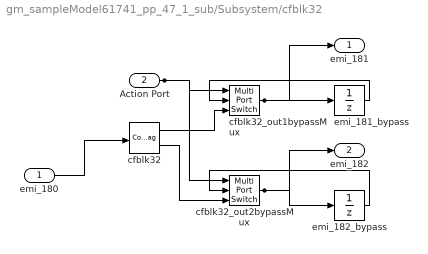
== system gm_sampleModel61741_pp_47_1_sub/Subsystem/cfblk32 ==
  emi_180 : Inport  OutDataTypeStr=uint8  PortDimensions=1  SampleTime=1
  Action Port : Inport  Port=2  OutDataTypeStr=boolean  SampleTime=1
  cfblk32 : ComplexToRealImag  SampleTime=1
  cfblk32_out1bypassMux : MultiPortSwitch  DataPortOrder=Zero-based contiguous  Inputs=2  zeroidx=on  OutDataTypeStr=uint8  SampleTime=1  SaturateOnIntegerOverflow=off  InputSameDT=off
  cfblk32_out2bypassMux : MultiPortSwitch  DataPortOrder=Zero-based contiguous  Inputs=2  zeroidx=on  OutDataTypeStr=uint8  SampleTime=1  SaturateOnIntegerOverflow=off  InputSameDT=off
  emi_181_bypass : UnitDelay  InitialCondition="fi(0,0,8,0,\"hex\",\"00\")"  SampleTime=1
  emi_182_bypass : UnitDelay  InitialCondition="fi(0,0,8,0,\"hex\",\"00\")"  SampleTime=1
  emi_181 : Outport  SampleTime=1  InitialOutput=0
  emi_182 : Outport  Port=2  SampleTime=1  InitialOutput=0
  wires:
  Action Port/1 -> cfblk32_out2bypassMux/1, cfblk32_out1bypassMux/1
  emi_180/1 -> cfblk32/1
  cfblk32/1 -> cfblk32_out1bypassMux/3
  cfblk32/2 -> cfblk32_out2bypassMux/3
  cfblk32_out1bypassMux/1 -> emi_181_bypass/1, emi_181/1
  emi_181_bypass/1 -> cfblk32_out1bypassMux/2
  cfblk32_out2bypassMux/1 -> emi_182_bypass/1, emi_182/1
  emi_182_bypass/1 -> cfblk32_out2bypassMux/2

== system gm_sampleModel61741_pp_47_1_sub/Subsystem/cfblk33 ==
  emi_352 : Inport  OutDataTypeStr=uint8  PortDimensions=1  SampleTime=1
  Action Port : Inport  Port=2  OutDataTypeStr=boolean  SampleTime=1
  cfblk33 : Abs  SampleTime=1  OutDataTypeStr=uint8  SaturateOnIntegerOverflow=off
  cfblk33_out1bypassMux : MultiPortSwitch  DataPortOrder=Zero-based contiguous  Inputs=2  zeroidx=on  OutDataTypeStr=uint8  SampleTime=1  SaturateOnIntegerOverflow=off  InputSameDT=off
  emi_353_bypass : UnitDelay  InitialCondition="fi(0,0,8,0,\"hex\",\"00\")"  SampleTime=1
  emi_353 : Outport  SampleTime=1  InitialOutput=0
  wires:
  Action Port/1 -> cfblk33_out1bypassMux/1
  emi_352/1 -> cfblk33/1
  cfblk33/1 -> cfblk33_out1bypassMux/3
  cfblk33_out1bypassMux/1 -> emi_353_bypass/1, emi_353/1
  emi_353_bypass/1 -> cfblk33_out1bypassMux/2

== system gm_sampleModel61741_pp_47_1_sub/Subsystem/cfblk34 ==
  u : Inport  OutDataTypeStr=uint8  SampleTime=1
  FixPt Constant : Constant  DisableCoverage=on  OutDataTypeStr=Inherit: Inherit via back propagation  SampleTime=-1
  FixPt Data Type Duplicate : DataTypeDuplicate  DisableCoverage=on  NumInputPorts=3
  FixPt Sum1 : Sum  OutDataTypeStr=Inherit: Inherit via back propagation  InputSameDT=on  LockScale=on
  y : Outport  SampleTime=1
  wires:
  u/1 -> FixPt Sum1/1, FixPt Data Type Duplicate/2
  FixPt Constant/1 -> FixPt Sum1/2, FixPt Data Type Duplicate/3
  FixPt Sum1/1 -> FixPt Data Type Duplicate/1, y/1

== system gm_sampleModel61741_pp_47_1_sub/Subsystem/cfblk38 ==
  u : Inport  OutDataTypeStr=uint8  SampleTime=1
  FixPt Constant : Constant  DisableCoverage=on  OutDataTypeStr=Inherit: Inherit via back propagation  SampleTime=-1
  FixPt Data Type Duplicate : DataTypeDuplicate  DisableCoverage=on  NumInputPorts=3
  FixPt Sum1 : Sum  OutDataTypeStr=Inherit: Inherit via back propagation  InputSameDT=on  LockScale=on
  y : Outport  SampleTime=1
  wires:
  u/1 -> FixPt Sum1/1, FixPt Data Type Duplicate/2
  FixPt Constant/1 -> FixPt Sum1/2, FixPt Data Type Duplicate/3
  FixPt Sum1/1 -> FixPt Data Type Duplicate/1, y/1
